simulink model "lab2_counterReset"  (R2024a)
settings: Solver=VariableStepAuto  StartTime=0.0  StopTime=10.0  RelTol=1e-3
libraries: simulink x1
settings Model: Creator=DELL  LastModifiedBy=DELL

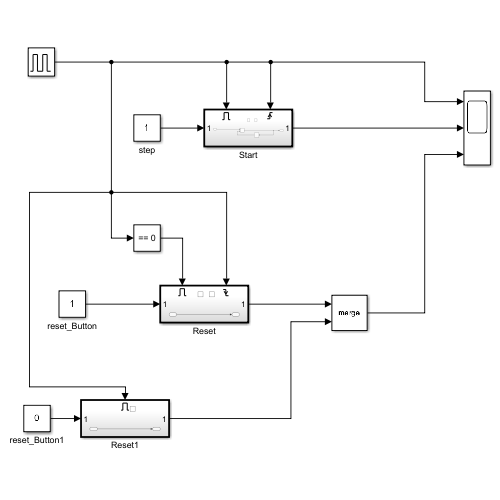
[thumbnail: Simulink's stored preview of the top-level diagram]
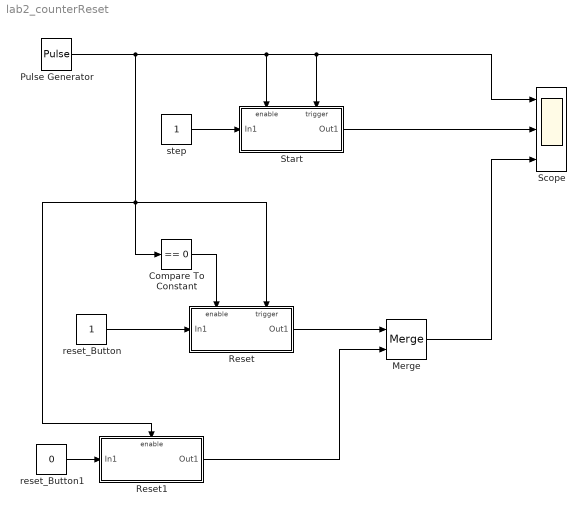
== system lab2_counterReset ==
  Compare To Constant : simulink/Logic and Bit Operations/Compare To Constant  relop===  const=0  OutDataTypeStr=boolean
  Merge : Merge
  Pulse Generator : DiscretePulseGenerator  PulseType=Time based  Period=1  PulseWidth=50
  Reset : Subsystem  TreatAsAtomicUnit=on
  Reset1 : Subsystem  TreatAsAtomicUnit=on
  Scope : Scope  NumInputPorts=3
  Start : Subsystem  TreatAsAtomicUnit=on
  reset_Button : Constant
  reset_Button1 : Constant  Value=0
  step : Constant
  wires:
  step/1 -> Start/1(In1)
  reset_Button/1 -> Reset/1(In1)
  Start/1(Out1) -> Scope/2
  Compare To Constant/1 -> Reset/Enable
  Pulse Generator/1 -> Start/Trigger, Scope/1, Start/Enable, Reset/Trigger, Reset1/Enable, Compare To Constant/1
  reset_Button1/1 -> Reset1/1(In1)
  Reset1/1(Out1) -> Merge/2
  Reset/1(Out1) -> Merge/1
  Merge/1 -> Scope/3

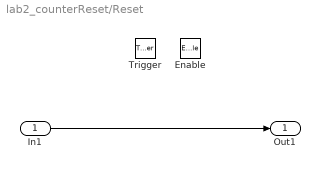
== system lab2_counterReset/Reset ==
  In1 : Inport
  Enable : EnablePort
  Trigger : TriggerPort  TriggerType=falling  VariantControl=(inherit)
  Out1 : Outport
  wires:
  In1/1 -> Out1/1

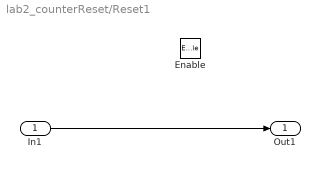
== system lab2_counterReset/Reset1 ==
  In1 : Inport
  Enable : EnablePort
  Out1 : Outport
  wires:
  In1/1 -> Out1/1

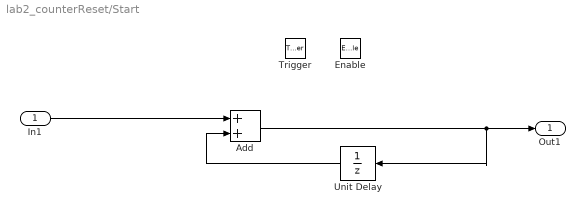
== system lab2_counterReset/Start ==
  In1 : Inport
  Enable : EnablePort
  Trigger : TriggerPort  VariantControl=(inherit)
  Add : Sum
  Unit Delay : UnitDelay  SampleTime=-1  HasFrameUpgradeWarning=on
  Out1 : Outport
  wires:
  In1/1 -> Add/1
  Add/1 -> Unit Delay/1, Out1/1
  Unit Delay/1 -> Add/2
